simulink model "BodeSim1"  (R2016a)
settings: Solver=ode45  StartTime=0.0  StopTime=5  MaxStep=0.00001  RelTol=1e-3
values from neighbouring files (symbols this model uses):
  T = 1/wc    (= 0.1)    [orden1_file.m]    (also in paraSimulink.m = 3.18309886184e-05)
  wi = wc/100    (= 314.159265359)    [paraSimulink.m]
  wz = 2*pi*28000    (= 175929.188601)    [paraSimulink.m]
settings Model: Creator=Gera  LastModifiedBy=itsaso
settings DataIOCC: LimitDataPoints=on  SaveFormat=Array  SignalLoggingSaveFormat=ModelDataLogs
settings OptimizationCC: ExpressionDepthLimit=2147483647  InitFltsAndDblsToZero=on
settings DebuggingCC: UnderspecifiedInitializationDetection=Classic  MergeDetectMultiDrivingBlocksExec=none  SolverPrmCheckMsg=warning  FcnCallInpInsideContextMsg=UseLocalSettings  StateNameClashWarn=warning
settings HardwareCC: ProdBitPerPointer=32  ProdLargestAtomicFloat=None  ProdIntDivRoundTo=Undefined  ProdEndianess=Unspecified  ProdWordSize=32  ProdHWDeviceType=32-bit Generic
settings ModelReferenceCC: PropagateSignalLabelsOutOfModel=off
settings GRTTargetCC: CombineOutputUpdateFcns=off  GRTInterface=on
settings ConfigComp: CovModelRefEnable=Off  CovSFcnEnable=off

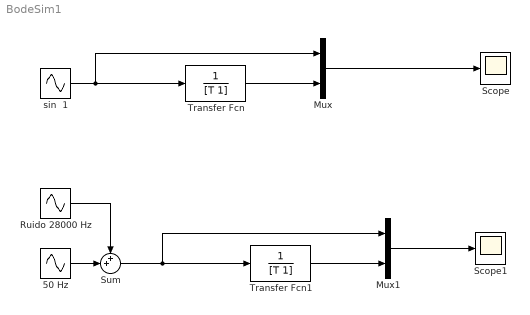
== system BodeSim1 ==
  50 Hz : Sin  Frequency=wi  SampleTime=0
  Mux : Mux  Inputs=2
  Mux1 : Mux  Inputs=2
  Ruido 28000 Hz : Sin  Amplitude=0.1  Frequency=wz  SampleTime=0
  Scope : Scope
  Scope1 : Scope
  Sum : Sum  Inputs=++|
  Transfer Fcn : TransferFcn  Denominator=[T 1]
  Transfer Fcn1 : TransferFcn  Denominator=[T 1]
  sin  1 : Sin  Frequency=wi  SampleTime=0
  wires:
  sin  1/1 -> Transfer Fcn/1, Mux/1
  Transfer Fcn/1 -> Mux/2
  Mux/1 -> Scope/1
  50 Hz/1 -> Sum/2
  Ruido 28000 Hz/1 -> Sum/1
  Transfer Fcn1/1 -> Mux1/2
  Mux1/1 -> Scope1/1
  Sum/1 -> Transfer Fcn1/1, Mux1/1
